simulink subsystem "ThermalModel"  (R2019b)
settings: Solver=VariableStepAuto  StartTime=0.0  StopTime=10.0  RelTol=1e-3
libraries: fl_lib x12, nesl_utility x6
settings Model: Creator=PcElettronicaDynamis  LastModifiedBy=PcElettronicaDynamis

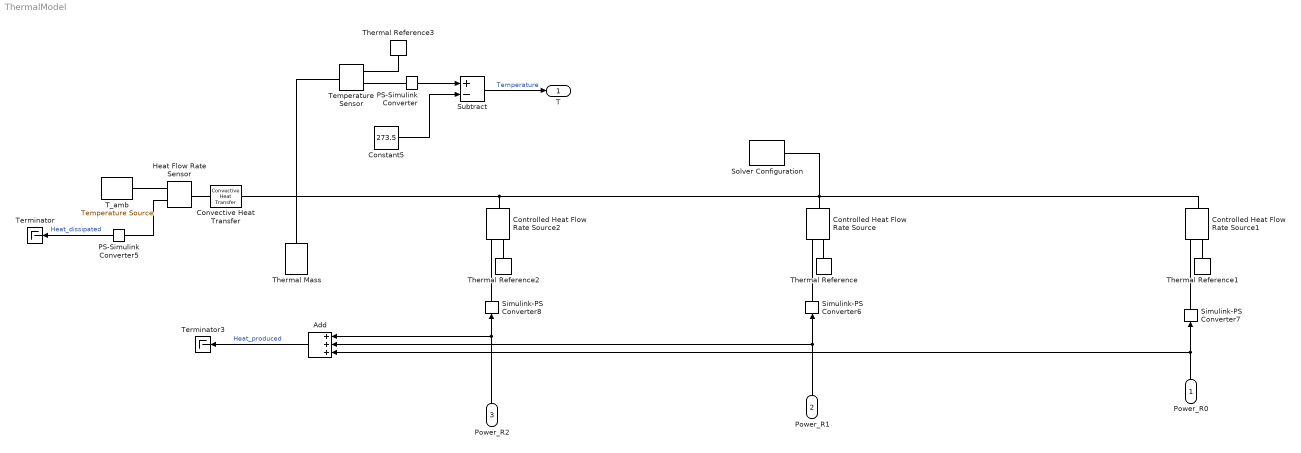
== system ThermalModel ==
  Power_R0 : Inport
  Power_R1 : Inport  Port=2
  Power_R2 : Inport  Port=3
  Add : Sum  Inputs=+++
  Constant5 : Constant  Value=273.5
  Controlled Heat Flow Rate Source : fl_lib/Thermal/Thermal Sources/Controlled Heat Flow Rate Source
      settings: SourceProductName=Simscape
  Controlled Heat Flow Rate Source1 : fl_lib/Thermal/Thermal Sources/Controlled Heat Flow Rate Source
      settings: SourceProductName=Simscape
  Controlled Heat Flow Rate Source2 : fl_lib/Thermal/Thermal Sources/Controlled Heat Flow Rate Source
      settings: SourceProductName=Simscape
  Convective Heat Transfer : fl_lib/Thermal/Thermal Elements/Convective Heat Transfer  area=18.35*pi*65+9*9*pi mm^2  heat_tr_coeff=15 W/(m^2 * K)  T_specify=off  T_priority=None  T=0 K  T_nominal_specify=off  T_nominal_unit=K  T_nominal_value=1  Q_specify=off  Q_priority=None  Q=0 W  Q_nominal_specify=off  Q_nominal_unit=W  Q_nominal_value=1
  Heat Flow Rate Sensor : fl_lib/Thermal/Thermal Sensors/Heat Flow Rate Sensor
      settings: SourceProductName=Simscape  SourceProductBaseCode=SS
  PS-Simulink Converter : nesl_utility/PS-Simulink Converter  PhysicalDomain=network_engine_domain  SubClassName=ps_output  LeftPortType=input  RightPortType=output  PseudoPeriodic=off  Frequencies=[]  Unit=1  AffineConversion=off
  PS-Simulink Converter5 : nesl_utility/PS-Simulink Converter  PhysicalDomain=network_engine_domain  SubClassName=ps_output  LeftPortType=input  RightPortType=output  PseudoPeriodic=off  Frequencies=[]  Unit=1  AffineConversion=off
  Simulink-PS Converter6 : nesl_utility/Simulink-PS Converter  PhysicalDomain=network_engine_domain  SubClassName=ps_input  LeftPortType=input  RightPortType=output  PseudoPeriodic=off  Frequencies=[]  NoiseDistribution=none  NoiseParameters=[]  Unit=1  AffineConversion=off  FilteringAndDerivatives=provide  SimscapeFilterOrder=1  InputFilterTimeConstant=0.001  UdotUserProvided=0
  Simulink-PS Converter7 : nesl_utility/Simulink-PS Converter  PhysicalDomain=network_engine_domain  SubClassName=ps_input  LeftPortType=input  RightPortType=output  PseudoPeriodic=off  Frequencies=[]  NoiseDistribution=none  NoiseParameters=[]  Unit=1  AffineConversion=off  FilteringAndDerivatives=provide  SimscapeFilterOrder=1  InputFilterTimeConstant=0.001  UdotUserProvided=0
  Simulink-PS Converter8 : nesl_utility/Simulink-PS Converter  PhysicalDomain=network_engine_domain  SubClassName=ps_input  LeftPortType=input  RightPortType=output  PseudoPeriodic=off  Frequencies=[]  NoiseDistribution=none  NoiseParameters=[]  Unit=1  AffineConversion=off  FilteringAndDerivatives=provide  SimscapeFilterOrder=1  InputFilterTimeConstant=0.001  UdotUserProvided=0
  Solver Configuration : nesl_utility/Solver Configuration  PhysicalDomain=network_engine_domain  SubClassName=solver  LeftPortType=input  RightPortType=generic  Tones=[]  Harmonics=[]  SimulateNoise=off  Profile=off  UseLocalSampling=off  EnableSwitchedLinearOptims=on  FrequencyDomain=off  UseCCode=off  RelTol=0.001  AbsTol=1e-06  MinStep=1e-09  ToWorkspace=off  RevertToSquareIcSolve=off  NumHomotopyIterations=100  PhasorMode=off  PhasorModeNumHarmonics=1  DoDC=on  ResidualTolerance=1e-09  UseLocalSolver=off  LocalSolverChoice=NE_BACKWARD_EULER_ADVANCER  LocalSolverSampleTime=0.001  DoFixedCost=off  MaxNonlinIter=3  MaxModeIter=2  LinearAlgebra=auto  EquationFormulation=NE_TIME_EF  DelaysMemoryBudget=1024  AutomaticFiltering=on  FilteringTimeConstant=0.001  PartitionStorageMethod=AS_NEEDED  PartitionMemoryBudget=1024  PartitionMethod=ROBUST
  Subtract : Sum  Inputs=+-
  T_amb : fl_lib/Thermal/Thermal Sources/Temperature Source  temperature=26 degC
      settings: SourceProductName=Simscape
  Temperature Sensor : fl_lib/Thermal/Thermal Sensors/Temperature Sensor
  Terminator : Terminator
  Terminator3 : Terminator
  Thermal Mass : fl_lib/Thermal/Thermal Elements/Thermal Mass  mass="46.4  g"  sp_heat=1000 J/kg/K  T_specify=on  T_priority=High  T=22 degC  T_nominal_specify=off  T_nominal_unit=K  T_nominal_value=1  Q_specify=off  Q_priority=None  Q=0 W  Q_nominal_specify=off  Q_nominal_unit=W  Q_nominal_value=1
  Thermal Reference{,1..3} (4 alike) : fl_lib/Thermal/Thermal Elements/Thermal Reference
  T : Outport
  wires:
  Constant5/1 -> Subtract/2
  PS-Simulink Converter5/1 -> Terminator/1  "Heat_dissipated"
  Power_R0/1 -> Simulink-PS Converter7/1, Add/3
  Subtract/1 -> T/1  "Temperature"
  PS-Simulink Converter/1 -> Subtract/1
  Add/1 -> Terminator3/1  "Heat_produced"
  Power_R1/1 -> Simulink-PS Converter6/1, Add/2
  Power_R2/1 -> Simulink-PS Converter8/1, Add/1
  connections:
  Controlled Heat Flow Rate Source/LConn1 -- Thermal Mass/LConn1 -- Convective Heat Transfer/LConn1 -- Temperature Sensor/LConn1 -- Controlled Heat Flow Rate Source2/LConn1 -- Controlled Heat Flow Rate Source1/LConn1 -- Solver Configuration/RConn1
  Convective Heat Transfer/RConn1 -- Heat Flow Rate Sensor/LConn1
  PS-Simulink Converter5/LConn1 -- Heat Flow Rate Sensor/RConn1
  Thermal Reference3/LConn1 -- Temperature Sensor/RConn1
  Thermal Reference/LConn1 -- Controlled Heat Flow Rate Source/RConn2
  Controlled Heat Flow Rate Source1/RConn1 -- Simulink-PS Converter7/RConn1
  Thermal Reference2/LConn1 -- Controlled Heat Flow Rate Source2/RConn2
  Simulink-PS Converter8/RConn1 -- Controlled Heat Flow Rate Source2/RConn1
  Simulink-PS Converter6/RConn1 -- Controlled Heat Flow Rate Source/RConn1
  Heat Flow Rate Sensor/RConn2 -- T_amb/LConn1
  PS-Simulink Converter/LConn1 -- Temperature Sensor/RConn2
  Thermal Reference1/LConn1 -- Controlled Heat Flow Rate Source1/RConn2
